simulink library "kelvinVoigtTether_cl"  (R2018b)
settings: Solver=VariableStepAuto  StartTime=0.0  StopTime=10.0  RelTol=1e-3
values from neighbouring files (symbols this model uses):
  G = 9.81    [kelvinVoightTether_ts.m]
  mass = 1000    [kelvinVoightTether_ts.m]
  rho_f = 1000    [kelvinVoightTether_ts.m]
undefined symbols (not defined in the file or in its folder): class_thr, n_ini_pos, n_ini_vel
libraries: tetherDragForceNEqual2_ul x1, tetherInternalForcesNEqual2_ul x1, tetherBuoyancyAndWeightNGreater2_ul x1, tetherDragForceNGreater2_ul x1, tetherInternalForcesNGreater2_ul x1
settings Model: Creator=Ayaz  LastModifiedBy=Ayaz

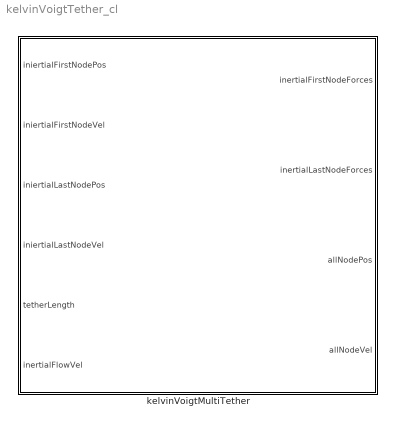
== system kelvinVoigtTether_cl ==
  kelvinVoigtMultiTether : Subsystem  TreatAsAtomicUnit=on  mask{rho_fluid=rho_f, grav=G, M=mass, tN=[class_thr.numNodes], tD=[class_thr.diameter], tRho=[class_thr.density], tE=[class_thr.youngsModulus], tZeta=[class_thr.dampingRatio], tCd=[class_thr.dragCoeff], iniR1_o=[class_thr.ini_R1_o], iniRn_o=[class_thr.ini_Rn_o], iniRi_o=n_ini_pos, iniVi_o=n_ini_vel}
      mask prompts: rho_fluid "Fluid Density"; grav "Gravitational acceleration"; M "Vehicle mass"; tN "Number of nodes"; tD "Tether diameters"; tRho "Tether densities"; tE "Tether Youngs Moduli"; tZeta "Tether damping ratios"; tCd "Tether drag coefficients"; iniR1_o "Initial first node positions"; iniRn_o "Initial last node positions"; iniRi_o "Initial nodal positions"; iniVi_o "Initial nodal velocities"
      mask init:
      | % initialization script
      | kelvinVoightTether_init_ts
      mask DialogControl Container3 Prompt: Environment
      mask DialogControl Container5 Prompt: Tethers
      mask DialogControl Container6 Prompt: Initial conditions

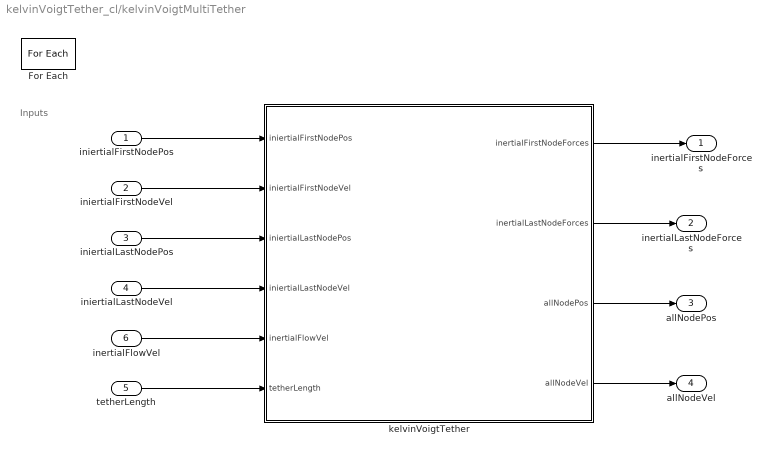
== system kelvinVoigtTether_cl/kelvinVoigtMultiTether ==
  note: Inputs
  iniertialFirstNodePos : Inport  Partition=on  PartitionDimension=2  PartitionWidth=1  PartitionOffset=0
  iniertialFirstNodeVel : Inport  Port=2  Partition=on  PartitionDimension=2  PartitionWidth=1  PartitionOffset=0
  iniertialLastNodePos : Inport  Port=3  Partition=on  PartitionDimension=2  PartitionWidth=1  PartitionOffset=0
  iniertialLastNodeVel : Inport  Port=4  Partition=on  PartitionDimension=2  PartitionWidth=1  PartitionOffset=0
  tetherLength : Inport  Port=5  Partition=on  PartitionDimension=2  PartitionWidth=1  PartitionOffset=0
  inertialFlowVel : Inport  Port=6
  For Each : ForEach  DisableCoverage=on  IterateSubsysMaskParameter=off,off,off,on,on,on,on,on,on,on,on,on,on  SubsysMaskParameterIterationDimension=1,1,1,2,2,2,2,2,2,2,2,3,3  SubsysMaskParameterIterationStepSize=1,1,1,1,1,1,1,1,1,2,2  IndexMode=One-based
  kelvinVoigtTether : Subsystem  VariantControlMode=Label  Variant=on  LabelModeActiveChoice=tetherNumNodeN_variant
  inertialFirstNodeForces : Outport  ConcatenationDimension=1
  inertialLastNodeForces : Outport  Port=2  ConcatenationDimension=1
  allNodePos : Outport  Port=3  ConcatenationDimension=1
  allNodeVel : Outport  Port=4  ConcatenationDimension=1
  wires:
  tetherLength/1 -> kelvinVoigtTether/6(tetherLength)
  iniertialFirstNodeVel/1 -> kelvinVoigtTether/2(iniertialFirstNodeVel)
  iniertialFirstNodePos/1 -> kelvinVoigtTether/1(iniertialFirstNodePos)
  iniertialLastNodeVel/1 -> kelvinVoigtTether/4(iniertialLastNodeVel)
  inertialFlowVel/1 -> kelvinVoigtTether/5(inertialFlowVel)
  iniertialLastNodePos/1 -> kelvinVoigtTether/3(iniertialLastNodePos)
  kelvinVoigtTether/1(inertialFirstNodeForces) -> inertialFirstNodeForces/1
  kelvinVoigtTether/2(inertialLastNodeForces) -> inertialLastNodeForces/1
  kelvinVoigtTether/3(allNodePos) -> allNodePos/1
  kelvinVoigtTether/4(allNodeVel) -> allNodeVel/1

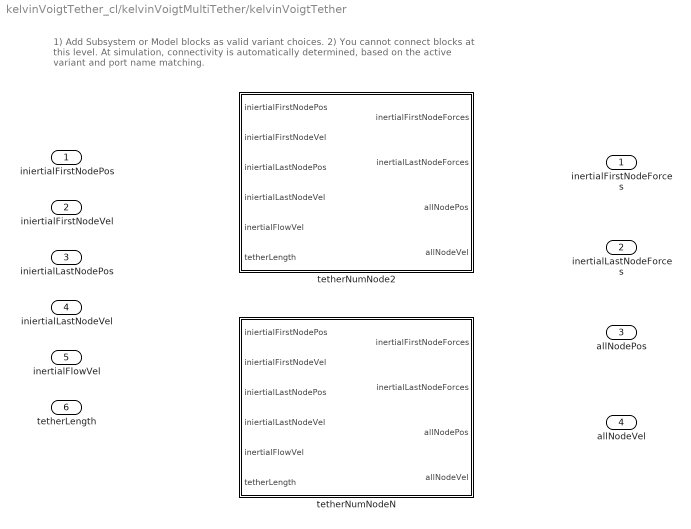
== system kelvinVoigtTether_cl/kelvinVoigtMultiTether/kelvinVoigtTether ==
  note: 1) Add Subsystem or Model blocks as valid variant choices.
      | 2) You cannot connect blocks at this level. At simulation, connectivity is automatically
      | determined, based on the active variant and port name matching.
  iniertialFirstNodePos : Inport
  iniertialFirstNodeVel : Inport  Port=2
  iniertialLastNodePos : Inport  Port=3
  iniertialLastNodeVel : Inport  Port=4
  inertialFlowVel : Inport  Port=5
  tetherLength : Inport  Port=6
  tetherNumNode2 : Subsystem  VariantControl=tetherNumNode2_variant
  tetherNumNodeN : Subsystem  VariantControl=tetherNumNodeN_variant
  inertialFirstNodeForces : Outport
  inertialLastNodeForces : Outport  Port=2
  allNodePos : Outport  Port=3
  allNodeVel : Outport  Port=4

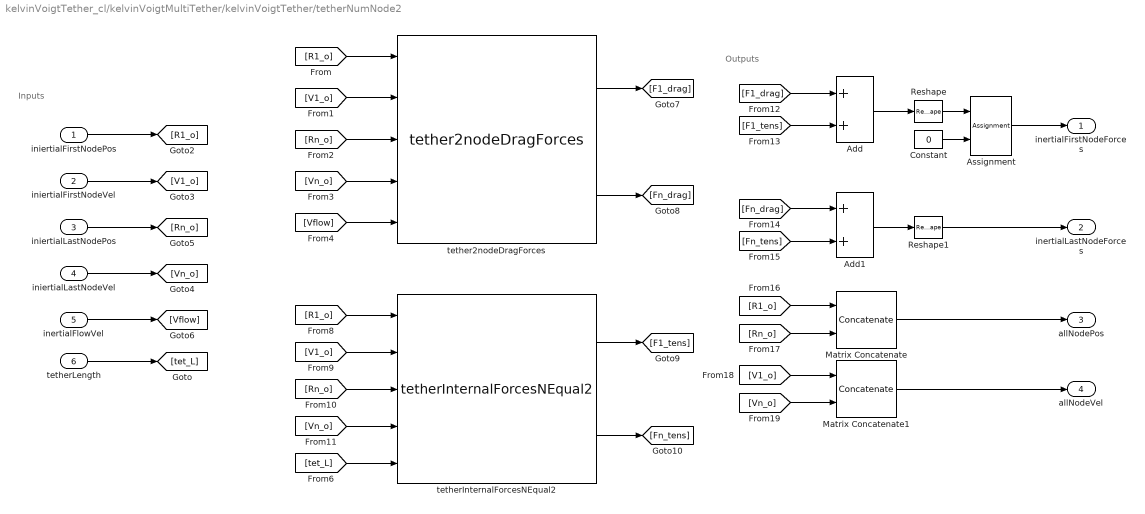
== system kelvinVoigtTether_cl/kelvinVoigtMultiTether/kelvinVoigtTether/tetherNumNode2 ==
  note: Outputs
  note: Inputs
  iniertialFirstNodePos : Inport
  iniertialFirstNodeVel : Inport  Port=2
  iniertialLastNodePos : Inport  Port=3
  iniertialLastNodeVel : Inport  Port=4
  inertialFlowVel : Inport  Port=5
  tetherLength : Inport  Port=6
  Add : Sum
  Add1 : Sum
  Assignment : Assignment  NumberOfDimensions=2  DiagnosticForDimensions=Warning  IndexOptions=Index vector (dialog),Index vector (dialog)  Indices=3,1  OutputSizes=1,1
  Constant : Constant  Value=0
  Matrix Concatenate : Concatenate  Mode=Multidimensional array  ConcatenateDimension=2
  Matrix Concatenate1 : Concatenate  Mode=Multidimensional array  ConcatenateDimension=2
  Reshape : Reshape  OutputDimensionality=Column vector (2-D)
  Reshape1 : Reshape  OutputDimensionality=Column vector (2-D)
  tether2nodeDragForces : tetherDragForceNEqual2_ul/tether2nodeDragForces  dia_t=tD  Cd=tCd  rho_fluid=rho_fluid
  tetherInternalForcesNEqual2 : tetherInternalForcesNEqual2_ul/tetherInternalForcesNEqual2  dia_t=tD  E=tE  mass=M  zeta=tZeta
  inertialFirstNodeForces : Outport
  inertialLastNodeForces : Outport  Port=2
  allNodePos : Outport  Port=3
  allNodeVel : Outport  Port=4
  wires:
  iniertialLastNodeVel/1 -> [Vn_o]
  inertialFlowVel/1 -> [Vflow]
  iniertialFirstNodePos/1 -> [R1_o]
  tetherLength/1 -> [tet_L]
  iniertialLastNodePos/1 -> [Rn_o]
  iniertialFirstNodeVel/1 -> [V1_o]
  [R1_o] -> tether2nodeDragForces/1
  [V1_o] -> tether2nodeDragForces/2
  [Rn_o] -> tether2nodeDragForces/3
  [Vn_o] -> tether2nodeDragForces/4
  [Vflow] -> tether2nodeDragForces/5
  [tet_L] -> tetherInternalForcesNEqual2/5
  [Vn_o] -> tetherInternalForcesNEqual2/4
  [Rn_o] -> tetherInternalForcesNEqual2/3
  [V1_o] -> tetherInternalForcesNEqual2/2
  [R1_o] -> tetherInternalForcesNEqual2/1
  tether2nodeDragForces/1 -> [F1_drag]
  tether2nodeDragForces/2 -> [Fn_drag]
  tetherInternalForcesNEqual2/2 -> [Fn_tens]
  tetherInternalForcesNEqual2/1 -> [F1_tens]
  [F1_drag] -> Add/1
  [F1_tens] -> Add/2
  [Fn_drag] -> Add1/1
  [Fn_tens] -> Add1/2
  [R1_o] -> Matrix Concatenate/1
  [Rn_o] -> Matrix Concatenate/2
  [V1_o] -> Matrix Concatenate1/1
  [Vn_o] -> Matrix Concatenate1/2
  Add/1 -> Reshape/1
  Add1/1 -> Reshape1/1
  Reshape1/1 -> inertialLastNodeForces/1
  Matrix Concatenate1/1 -> allNodeVel/1
  Matrix Concatenate/1 -> allNodePos/1
  Reshape/1 -> Assignment/1
  Assignment/1 -> inertialFirstNodeForces/1
  Constant/1 -> Assignment/2

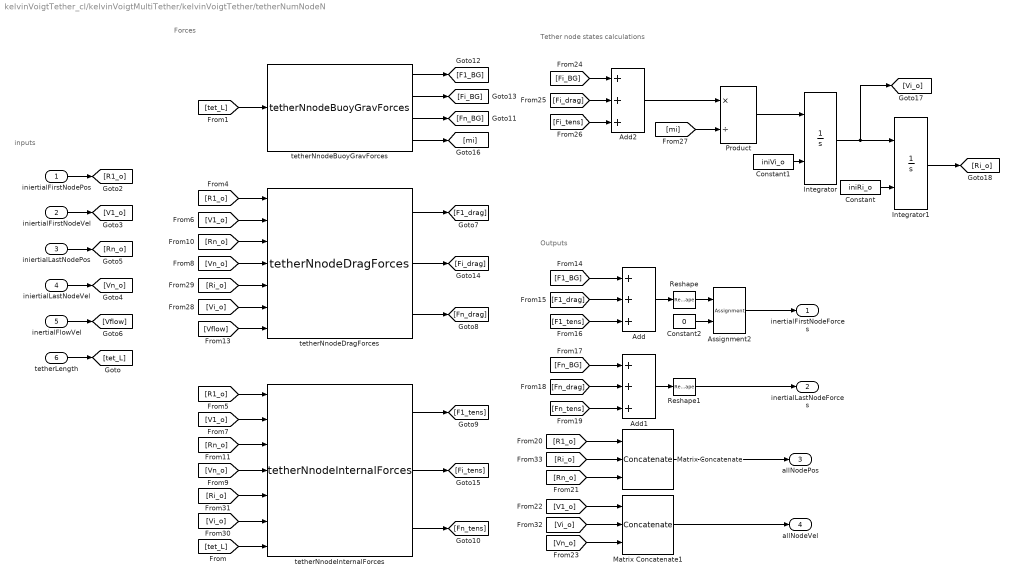
== system kelvinVoigtTether_cl/kelvinVoigtMultiTether/kelvinVoigtTether/tetherNumNodeN ==
  note: Tether node states calculations
  note: Outputs
  note: Forces
  note: inputs
  iniertialFirstNodePos : Inport
  iniertialFirstNodeVel : Inport  Port=2
  iniertialLastNodePos : Inport  Port=3
  iniertialLastNodeVel : Inport  Port=4
  inertialFlowVel : Inport  Port=5
  tetherLength : Inport  Port=6
  Add : Sum  Inputs=+++
  Add1 : Sum  Inputs=+++
  Add2 : Sum  Inputs=+++
  Assignment2 : Assignment  NumberOfDimensions=2  DiagnosticForDimensions=Warning  IndexOptions=Index vector (dialog),Index vector (dialog)  Indices=3,1  OutputSizes=1,1
  Constant : Constant  Value=iniRi_o  VectorParams1D=off
  Constant1 : Constant  Value=iniVi_o  VectorParams1D=off
  Constant2 : Constant  Value=0
  Integrator : Integrator  InitialConditionSource=external
  Integrator1 : Integrator  InitialConditionSource=external
  Matrix Concatenate : Concatenate  NumInputs=3  Mode=Multidimensional array  ConcatenateDimension=2
  Matrix Concatenate1 : Concatenate  NumInputs=3  Mode=Multidimensional array  ConcatenateDimension=2
  Product : Product  Inputs=*/
  Reshape : Reshape  OutputDimensionality=Column vector (2-D)
  Reshape1 : Reshape  OutputDimensionality=Column vector (2-D)
  tetherNnodeBuoyGravForces : tetherBuoyancyAndWeightNGreater2_ul/tetherNnodeBuoyGravForces  N=tN  dia_t=tD  rho_fluid=rho_fluid  rho_tether=tRho  g=grav
  tetherNnodeDragForces : tetherDragForceNGreater2_ul/tetherNnodeDragForces  N=tN  dia_t=tD  Cd=tCd  rho_fluid=rho_fluid
  tetherNnodeInternalForces : tetherInternalForcesNGreater2_ul/tetherNnodeInternalForces  N=tN  dia_t=tD  E=tE  mass=M  zeta=tZeta
  inertialFirstNodeForces : Outport
  inertialLastNodeForces : Outport  Port=2
  allNodePos : Outport  Port=3
  allNodeVel : Outport  Port=4
  wires:
  tetherLength/1 -> [tet_L]
  [tet_L] -> tetherNnodeInternalForces/7
  [tet_L] -> tetherNnodeBuoyGravForces/1
  iniertialFirstNodePos/1 -> [R1_o]
  [R1_o] -> tetherNnodeDragForces/1
  [R1_o] -> tetherNnodeInternalForces/1
  iniertialFirstNodeVel/1 -> [V1_o]
  [V1_o] -> tetherNnodeDragForces/2
  [V1_o] -> tetherNnodeInternalForces/2
  iniertialLastNodeVel/1 -> [Vn_o]
  [Vn_o] -> tetherNnodeDragForces/4
  [Vn_o] -> tetherNnodeInternalForces/4
  iniertialLastNodePos/1 -> [Rn_o]
  [Rn_o] -> tetherNnodeDragForces/3
  [Rn_o] -> tetherNnodeInternalForces/3
  inertialFlowVel/1 -> [Vflow]
  [Vflow] -> tetherNnodeDragForces/7
  tetherNnodeDragForces/1 -> [F1_drag]
  tetherNnodeInternalForces/1 -> [F1_tens]
  tetherNnodeDragForces/3 -> [Fn_drag]
  tetherNnodeInternalForces/3 -> [Fn_tens]
  tetherNnodeBuoyGravForces/3 -> [Fn_BG]
  tetherNnodeBuoyGravForces/1 -> [F1_BG]
  tetherNnodeBuoyGravForces/2 -> [Fi_BG]
  tetherNnodeDragForces/2 -> [Fi_drag]
  tetherNnodeInternalForces/2 -> [Fi_tens]
  [F1_BG] -> Add/1
  [F1_drag] -> Add/2
  [F1_tens] -> Add/3
  Add/1 -> Reshape/1
  [Fn_BG] -> Add1/1
  [Fn_tens] -> Add1/3
  Add1/1 -> Reshape1/1
  [Fn_drag] -> Add1/2
  [R1_o] -> Matrix Concatenate/1
  [V1_o] -> Matrix Concatenate1/1
  Matrix Concatenate/1 -> allNodePos/1
  Matrix Concatenate1/1 -> allNodeVel/1
  [Rn_o] -> Matrix Concatenate/3
  [Vn_o] -> Matrix Concatenate1/3
  [Fi_drag] -> Add2/2
  [Fi_tens] -> Add2/3
  [Fi_BG] -> Add2/1
  tetherNnodeBuoyGravForces/4 -> [mi]
  Add2/1 -> Product/1
  [mi] -> Product/2
  Product/1 -> Integrator/1
  Integrator/1 -> [Vi_o], Integrator1/1
  Integrator1/1 -> [Ri_o]
  [Vi_o] -> tetherNnodeDragForces/6
  [Ri_o] -> tetherNnodeDragForces/5
  [Vi_o] -> tetherNnodeInternalForces/6
  [Ri_o] -> tetherNnodeInternalForces/5
  [Vi_o] -> Matrix Concatenate1/2
  [Ri_o] -> Matrix Concatenate/2
  Constant2/1 -> Assignment2/2
  Reshape/1 -> Assignment2/1
  Reshape1/1 -> inertialLastNodeForces/1
  Assignment2/1 -> inertialFirstNodeForces/1
  Constant/1 -> Integrator1/2
  Constant1/1 -> Integrator/2
